simulink model "obstaculo1_pibit_2025"  (R2025a)
settings: Solver=ode45  StartTime=0.0  StopTime=30  RelTol=1e-3
values from neighbouring files (symbols this model uses):
  a_Ax = 0.070    (= 0.07)    [parametros_suspensao_completo_pibit_final.m]
  entre_eixos = 0.184356    [parametros_suspensao_completo_pibit_final.m]
  Hmax = 10/100    (= 0.1)    [parametros_suspensao_completo_pibit_final.m]
  Lqm = 3,7    [parametros_suspensao_completo_pibit_final.m]
  Vv = 5    [parametros_suspensao_completo_pibit_final.m]
undefined symbols (not defined in the file or in its folder): t_reto_diant, Xcg

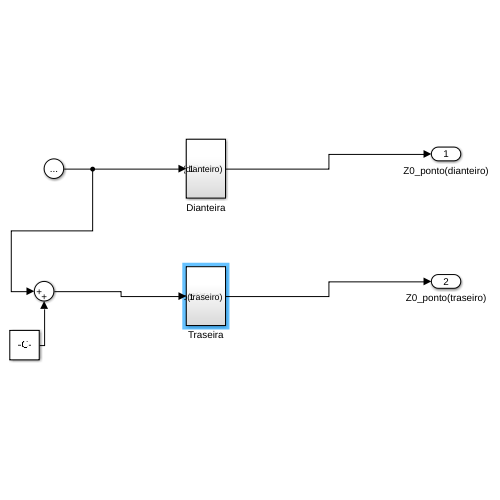
[thumbnail: Simulink's stored preview of the top-level diagram]
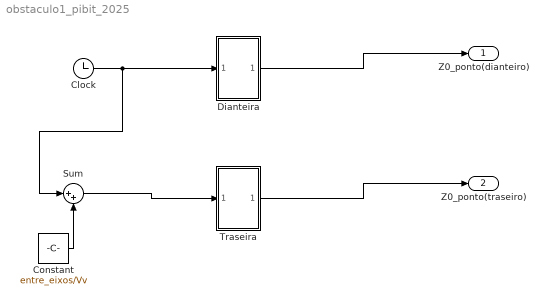
== system obstaculo1_pibit_2025 ==
  Clock : Clock
  Constant : Constant  Value=entre_eixos/Vv
  Dianteira : Subsystem
  Sum : Sum  Inputs=|++
  Traseira : Subsystem
  Z0_ponto(dianteiro) : Outport
  Z0_ponto(traseiro) : Outport  Port=2
  wires:
  Dianteira/1(Z0_ponto(dianteiro)) -> Z0_ponto(dianteiro)/1
  Traseira/1(Z0_ponto(traseiro)) -> Z0_ponto(traseiro)/1
  Clock/1 -> Sum/1, Dianteira/1(In1)
  Sum/1 -> Traseira/1(In1)
  Constant/1 -> Sum/2

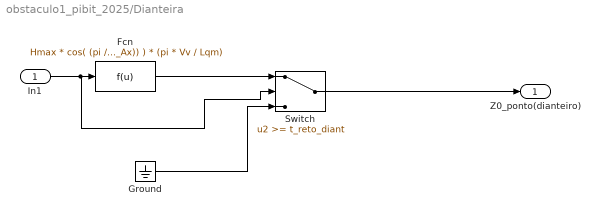
== system obstaculo1_pibit_2025/Dianteira ==
  In1 : Inport
  Fcn : Fcn  Expr=Hmax * cos( (pi / Lqm) * (Vv * u - (Xcg - a_Ax)) ) * (pi * Vv / Lqm)
  Ground : Ground
  Switch : Switch  Threshold=t_reto_diant  SaturateOnIntegerOverflow=off  InputSameDT=off
  Z0_ponto(dianteiro) : Outport
  wires:
  Switch/1 -> Z0_ponto(dianteiro)/1
  In1/1 -> Fcn/1, Switch/2
  Ground/1 -> Switch/3
  Fcn/1 -> Switch/1

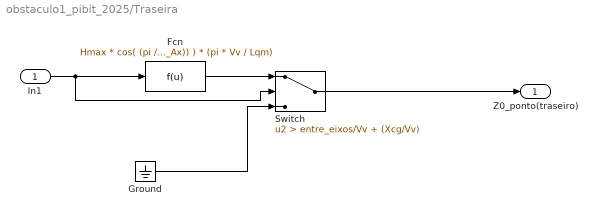
== system obstaculo1_pibit_2025/Traseira ==
  In1 : Inport
  Fcn : Fcn  Expr=Hmax * cos( (pi / Lqm) * (Vv * u - (Xcg - a_Ax)) ) * (pi * Vv / Lqm)
  Ground : Ground
  Switch : Switch  Criteria=u2 > Threshold  Threshold=entre_eixos/Vv + (Xcg/Vv)  SaturateOnIntegerOverflow=off  InputSameDT=off
  Z0_ponto(traseiro) : Outport
  wires:
  Switch/1 -> Z0_ponto(traseiro)/1
  In1/1 -> Fcn/1, Switch/2
  Ground/1 -> Switch/3
  Fcn/1 -> Switch/1
